simulink model "three_back_forth"  (R2023a)
settings: Solver=ode5  StartTime=0.0  StopTime=inf  FixedStep=0.001  RelTol=1e-3
undefined symbols (not defined in the file or in its folder): LF
libraries: instrumentseriallib x9, sldrtlib x1
settings Model: Creator=DELL  LastModifiedBy=DELL
settings HardwareCC: ProdBitPerLong=64  ProdHWDeviceType=Intel->x86-64 (Linux 64)
settings ModelReferenceCC: EnableRefExpFcnMdlSchedulingChecks=on
settings RTWCC: Description=Simulink Desktop Real-Time  SystemTargetFile=sldrt.tlc  TemplateMakefile=sldrt.tmf  RTWCompilerOptimization=on
settings CodeAppCC: MaxIdLength=95
settings SimulinkDesktopRealTimeCC: TargetLibSuffix=_sldrt.a  TargetPreCompLibLocation=C:\Program Files\MATLAB\R2023a\toolbox\sldrt\lib\win64

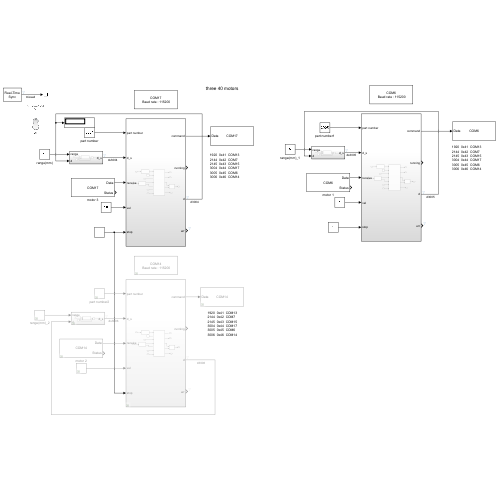
[thumbnail: Simulink's stored preview of the top-level diagram]
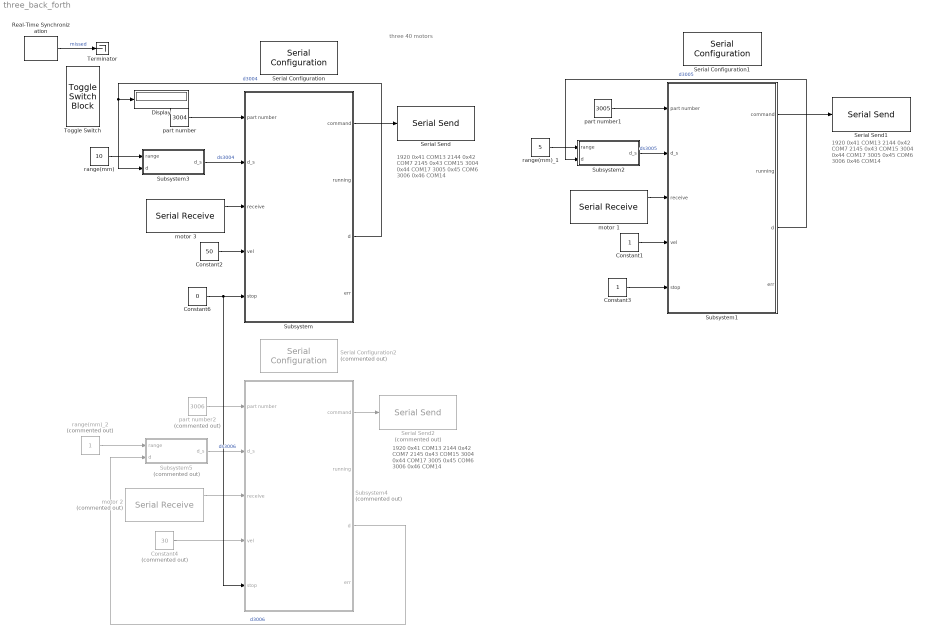
== system three_back_forth ==
  note: 1920  0x41  COM13
      | 2144  0x42  COM7
      | 2145  0x43  COM15
      | 3004  0x44  COM17
      | 3005  0x45  COM6
      | 3006  0x46  COM14
  note: 1920  0x41  COM13
      | 2144  0x42  COM7
      | 2145  0x43  COM15
      | 3004  0x44  COM17
      | 3005  0x45  COM6
      | 3006  0x46  COM14
  note: 1920  0x41  COM13
      | 2144  0x42  COM7
      | 2145  0x43  COM15
      | 3004  0x44  COM17
      | 3005  0x45  COM6
      | 3006  0x46  COM14
  note: three 40 motors
  Constant1 : Constant
  Constant2 : Constant  Value=50
  Constant3 : Constant
  Constant4 : Constant  Commented=on  Value=30
  Constant6 : Constant  Value=0
  Display : Display
  Real-Time Synchronization : sldrtlib/Real-Time Synchronization  SampleTime=0.1  MaxMissedTicks=10  ShowMissedTicks=on  YieldWhenWaiting=off
  Serial Configuration : instrumentseriallib/Serial Configuration  Priority=-200000  PortSel=COM17  Port=COM17  ComPort=COM17  BaudRate=115200  DataBits=8  Parity=none  StopBits=1  ByteOrder=little-endian  FlowControl=none  Timeout=10  SimulateUsing=Interpreted execution  BlockInModel=on  aMode=1
  Serial Configuration1 : instrumentseriallib/Serial Configuration  Priority=-200000  PortSel=COM6  Port=COM6  ComPort=COM6  BaudRate=115200  DataBits=8  Parity=none  StopBits=1  ByteOrder=little-endian  FlowControl=none  Timeout=10  SimulateUsing=Interpreted execution  BlockInModel=on  aMode=1
  Serial Configuration2 : instrumentseriallib/Serial Configuration  Priority=-200000  Commented=on  PortSel=COM14  Port=COM14  ComPort=COM14  BaudRate=115200  DataBits=8  Parity=none  StopBits=1  ByteOrder=little-endian  FlowControl=none  Timeout=10  SimulateUsing=Interpreted execution  BlockInModel=on  aMode=1
  Serial Send : instrumentseriallib/Serial Send  Priority=1  PortSel=COM17  Port=COM17  ComPort=COM17  Header=[]  Terminator=<none>  CustomTerminator=[]  EnableBlockingMode=off  SimulateUsing=Interpreted execution  BlockInModel=on  aMode=1
  Serial Send1 : instrumentseriallib/Serial Send  Priority=1  PortSel=COM6  Port=COM6  ComPort=COM6  Header=[]  Terminator=<none>  CustomTerminator=[]  EnableBlockingMode=off  SimulateUsing=Interpreted execution  BlockInModel=on  aMode=1
  Serial Send2 : instrumentseriallib/Serial Send  Priority=1  Commented=on  PortSel=COM14  Port=COM14  ComPort=COM14  Header=[]  Terminator=<none>  CustomTerminator=[]  EnableBlockingMode=off  SimulateUsing=Interpreted execution  BlockInModel=on  aMode=1
  Subsystem : Subsystem
  Subsystem1 : Subsystem
  Subsystem2 : Subsystem
  Subsystem3 : Subsystem
  Subsystem4 : Subsystem  Commented=on
  Subsystem5 : Subsystem  Commented=on
  Terminator : Terminator
  Toggle Switch : ToggleSwitchBlock
      settings: Values={{'Off', 'On'}, [0 1]}
  motor 1 : instrumentseriallib/Serial Receive  Priority=1  PortSel=COM6  Port=COM6  ComPort=COM6  DataType=uint8  SaveDataType=uint8  ToggleHeader=off  Header=[]  ToggleTerminator=on  Terminator=LF ('\n')  CustomTerminator=[]  InputFormat=Column major  ToggleDataSize=on  DataSize=[1 7]  EnableBlockingMode=off  ActionDataUnavailable=Output last received value  ActionWhenDataUnavailable=Output last received value  CustomValue=0  SampleTime=0.01  SimulateUsing=Interpreted execution  BlockInModel=on  aMode=1
  motor 2 : instrumentseriallib/Serial Receive  Priority=1  Commented=on  PortSel=COM14  Port=COM14  ComPort=COM14  DataType=uint8  SaveDataType=uint8  ToggleHeader=off  Header=[]  ToggleTerminator=on  Terminator=LF ('\n')  CustomTerminator=[]  InputFormat=Column major  ToggleDataSize=on  DataSize=[1 7]  EnableBlockingMode=off  ActionDataUnavailable=Output last received value  ActionWhenDataUnavailable=Output last received value  CustomValue=0  SampleTime=0.01  SimulateUsing=Interpreted execution  BlockInModel=on  aMode=1
  motor 3 : instrumentseriallib/Serial Receive  Priority=1  PortSel=COM17  Port=COM17  ComPort=COM17  DataType=uint8  SaveDataType=uint8  ToggleHeader=off  Header=[]  ToggleTerminator=on  Terminator=LF ('\n')  CustomTerminator=[]  InputFormat=Column major  ToggleDataSize=on  DataSize=[1 7]  EnableBlockingMode=off  ActionDataUnavailable=Output last received value  ActionWhenDataUnavailable=Output last received value  CustomValue=0  SampleTime=0.01  SimulateUsing=Interpreted execution  BlockInModel=on  aMode=1
  part number : Constant  Value=3004
  part number1 : Constant  Value=3005
  part number2 : Constant  Commented=on  Value=3006
  range(mm) : Constant  Value=10
  range(mm)_1 : Constant  Value=5
  range(mm)_2 : Constant  Commented=on
  wires:
  range(mm)/1 -> Subsystem3/1(range)
  part number/1 -> Subsystem/1(part number)
  Subsystem3/1(d_s) -> Subsystem/2(d_s)  "ds3004"
  motor 3/1 -> Subsystem/3(receive)
  Subsystem/1(command) -> Serial Send/1
  Subsystem/3(d) -> Display/1, Subsystem3/2(d)  "d3004"
  Constant2/1 -> Subsystem/4(vel)
  Subsystem1/1(command) -> Serial Send1/1
  Constant1/1 -> Subsystem1/4(vel)
  part number1/1 -> Subsystem1/1(part number)
  motor 1/1 -> Subsystem1/3(receive)
  Subsystem2/1(d_s) -> Subsystem1/2(d_s)  "ds3005"
  range(mm)_1/1 -> Subsystem2/1(range)
  Subsystem1/3(d) -> Subsystem2/2(d)  "d3005"
  Subsystem4/1(command) -> Serial Send2/1
  Constant4/1 -> Subsystem4/4(vel)
  part number2/1 -> Subsystem4/1(part number)
  motor 2/1 -> Subsystem4/3(receive)
  Subsystem5/1(d_s) -> Subsystem4/2(d_s)  "ds3006"
  range(mm)_2/1 -> Subsystem5/1(range)
  Subsystem4/3(d) -> Subsystem5/2(d)  "d3006"
  Real-Time Synchronization/1 -> Terminator/1  "missed"
  Constant6/1 -> Subsystem4/5(stop), Subsystem/5(stop)
  Constant3/1 -> Subsystem1/5(stop)

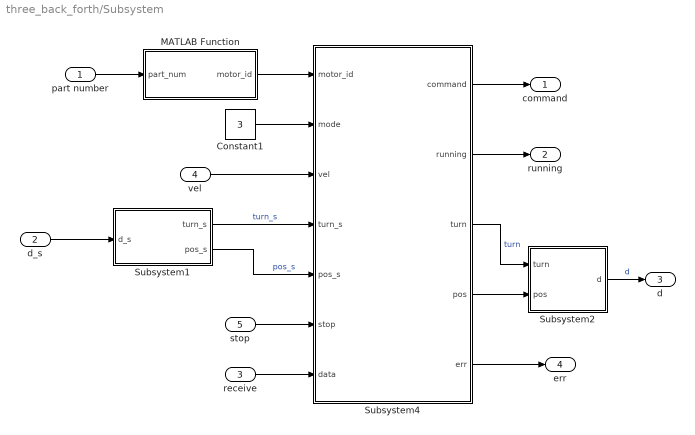
== system three_back_forth/Subsystem ==
  part number : Inport
  d_s : Inport  Port=2
  receive : Inport  Port=3
  vel : Inport  Port=4
  stop : Inport  Port=5
  Constant1 : Constant  Value=3
  MATLAB Function : MATLAB Function  TreatAsAtomicUnit=on
  Subsystem1 : Subsystem
  Subsystem2 : Subsystem
  Subsystem4 : Subsystem
  command : Outport
  running : Outport  Port=2
  d : Outport  Port=3
  err : Outport  Port=4
  wires:
  Constant1/1 -> Subsystem4/2(mode)
  Subsystem4/2(running) -> running/1
  Subsystem1/1(turn_s) -> Subsystem4/4(turn_s)  "turn_s"
  Subsystem1/2(pos_s) -> Subsystem4/5(pos_s)  "pos_s"
  Subsystem4/3(turn) -> Subsystem2/1(turn)  "turn"
  Subsystem4/1(command) -> command/1
  Subsystem4/4(pos) -> Subsystem2/2(pos)
  vel/1 -> Subsystem4/3(vel)
  stop/1 -> Subsystem4/6(stop)
  receive/1 -> Subsystem4/7(data)
  part number/1 -> MATLAB Function/1(part_num)
  Subsystem2/1(d) -> d/1  "d"
  d_s/1 -> Subsystem1/1(d_s)
  Subsystem4/5(err) -> err/1
  MATLAB Function/1(motor_id) -> Subsystem4/1(motor_id)

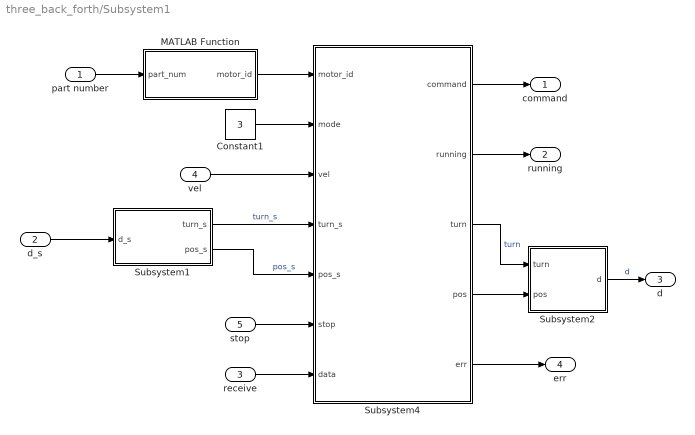
== system three_back_forth/Subsystem1 ==
  part number : Inport
  d_s : Inport  Port=2
  receive : Inport  Port=3
  vel : Inport  Port=4
  stop : Inport  Port=5
  Constant1 : Constant  Value=3
  MATLAB Function : MATLAB Function  TreatAsAtomicUnit=on
  Subsystem1 : Subsystem
  Subsystem2 : Subsystem
  Subsystem4 : Subsystem
  command : Outport
  running : Outport  Port=2
  d : Outport  Port=3
  err : Outport  Port=4
  wires:
  Constant1/1 -> Subsystem4/2(mode)
  Subsystem4/2(running) -> running/1
  Subsystem1/1(turn_s) -> Subsystem4/4(turn_s)  "turn_s"
  Subsystem1/2(pos_s) -> Subsystem4/5(pos_s)  "pos_s"
  Subsystem4/3(turn) -> Subsystem2/1(turn)  "turn"
  Subsystem4/1(command) -> command/1
  Subsystem4/4(pos) -> Subsystem2/2(pos)
  vel/1 -> Subsystem4/3(vel)
  stop/1 -> Subsystem4/6(stop)
  receive/1 -> Subsystem4/7(data)
  part number/1 -> MATLAB Function/1(part_num)
  Subsystem2/1(d) -> d/1  "d"
  d_s/1 -> Subsystem1/1(d_s)
  Subsystem4/5(err) -> err/1
  MATLAB Function/1(motor_id) -> Subsystem4/1(motor_id)

== system three_back_forth/Subsystem2 ==
  range : Inport
  d : Inport  Port=2
  Constant : Constant  Value=0.001
  MATLAB System : MATLABSystem  System=toggle_system  SimulateUsing=Code generation
      mask Type: toggle_system
      mask Display:
      | disp('toggle_system');
      | port_label('input',1,'range');
      | port_label('input',2,'d');
      | port_label('input',3,'margin');
      | port_label('output',1,'toggle');
  Product : Product
  d_s : Outport
  wires:
  d/1 -> MATLAB System/2
  range/1 -> Product/2, MATLAB System/1
  MATLAB System/1 -> Product/1
  Product/1 -> d_s/1
  Constant/1 -> MATLAB System/3

== system three_back_forth/Subsystem3 ==
  range : Inport
  d : Inport  Port=2
  Constant : Constant  Value=0.001
  MATLAB System : MATLABSystem  System=toggle_system  SimulateUsing=Code generation
      mask Type: toggle_system
      mask Display:
      | disp('toggle_system');
      | port_label('input',1,'range');
      | port_label('input',2,'d');
      | port_label('input',3,'margin');
      | port_label('output',1,'toggle');
  Product : Product
  d_s : Outport
  wires:
  d/1 -> MATLAB System/2
  range/1 -> Product/2, MATLAB System/1
  MATLAB System/1 -> Product/1
  Product/1 -> d_s/1
  Constant/1 -> MATLAB System/3

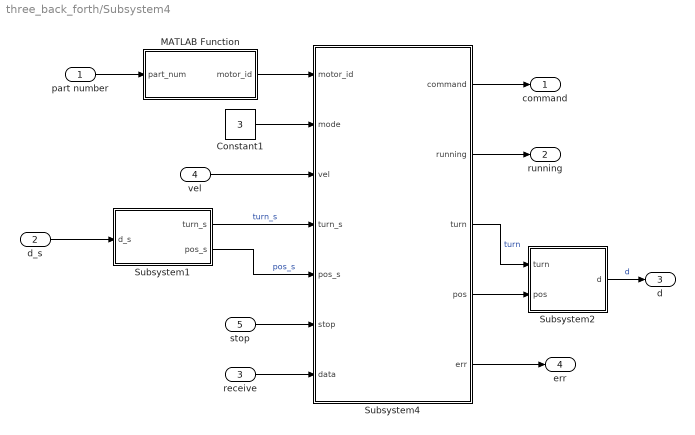
== system three_back_forth/Subsystem4 ==
  part number : Inport
  d_s : Inport  Port=2
  receive : Inport  Port=3
  vel : Inport  Port=4
  stop : Inport  Port=5
  Constant1 : Constant  Value=3
  MATLAB Function : MATLAB Function  TreatAsAtomicUnit=on
  Subsystem1 : Subsystem
  Subsystem2 : Subsystem
  Subsystem4 : Subsystem
  command : Outport
  running : Outport  Port=2
  d : Outport  Port=3
  err : Outport  Port=4
  wires:
  Constant1/1 -> Subsystem4/2(mode)
  Subsystem4/2(running) -> running/1
  Subsystem1/1(turn_s) -> Subsystem4/4(turn_s)  "turn_s"
  Subsystem1/2(pos_s) -> Subsystem4/5(pos_s)  "pos_s"
  Subsystem4/3(turn) -> Subsystem2/1(turn)  "turn"
  Subsystem4/1(command) -> command/1
  Subsystem4/4(pos) -> Subsystem2/2(pos)
  vel/1 -> Subsystem4/3(vel)
  stop/1 -> Subsystem4/6(stop)
  receive/1 -> Subsystem4/7(data)
  part number/1 -> MATLAB Function/1(part_num)
  Subsystem2/1(d) -> d/1  "d"
  d_s/1 -> Subsystem1/1(d_s)
  Subsystem4/5(err) -> err/1
  MATLAB Function/1(motor_id) -> Subsystem4/1(motor_id)

== system three_back_forth/Subsystem5 ==
  range : Inport
  d : Inport  Port=2
  Constant : Constant  Value=0.001
  MATLAB System : MATLABSystem  System=toggle_system  SimulateUsing=Code generation
      mask Type: toggle_system
      mask Display:
      | disp('toggle_system');
      | port_label('input',1,'range');
      | port_label('input',2,'d');
      | port_label('input',3,'margin');
      | port_label('output',1,'toggle');
  Product : Product
  d_s : Outport
  wires:
  d/1 -> MATLAB System/2
  range/1 -> Product/2, MATLAB System/1
  MATLAB System/1 -> Product/1
  Product/1 -> d_s/1
  Constant/1 -> MATLAB System/3

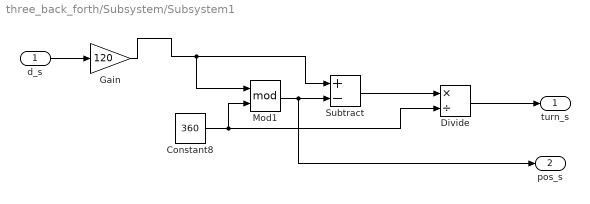
== system three_back_forth/Subsystem/Subsystem1 ==
  d_s : Inport
  Constant8 : Constant  Value=360
  Divide : Product  Inputs=*/
  Gain : Gain  Gain=120
  Mod1 : Math  Operator=mod
  Subtract : Sum  Inputs=+-
  turn_s : Outport
  pos_s : Outport  Port=2
  wires:
  Constant8/1 -> Divide/2, Mod1/2
  Gain/1 -> Subtract/1, Mod1/1
  Mod1/1 -> pos_s/1, Subtract/2
  Subtract/1 -> Divide/1
  Divide/1 -> turn_s/1
  d_s/1 -> Gain/1

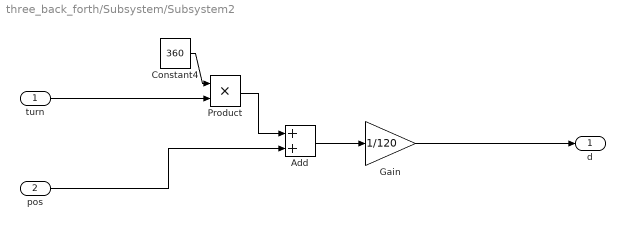
== system three_back_forth/Subsystem/Subsystem2 ==
  turn : Inport
  pos : Inport  Port=2
  Add : Sum
  Constant4 : Constant  Value=360
  Gain : Gain  Gain=1/120
  Product : Product
  d : Outport
  wires:
  turn/1 -> Product/2
  Add/1 -> Gain/1
  Constant4/1 -> Product/1
  Product/1 -> Add/1
  Gain/1 -> d/1
  pos/1 -> Add/2

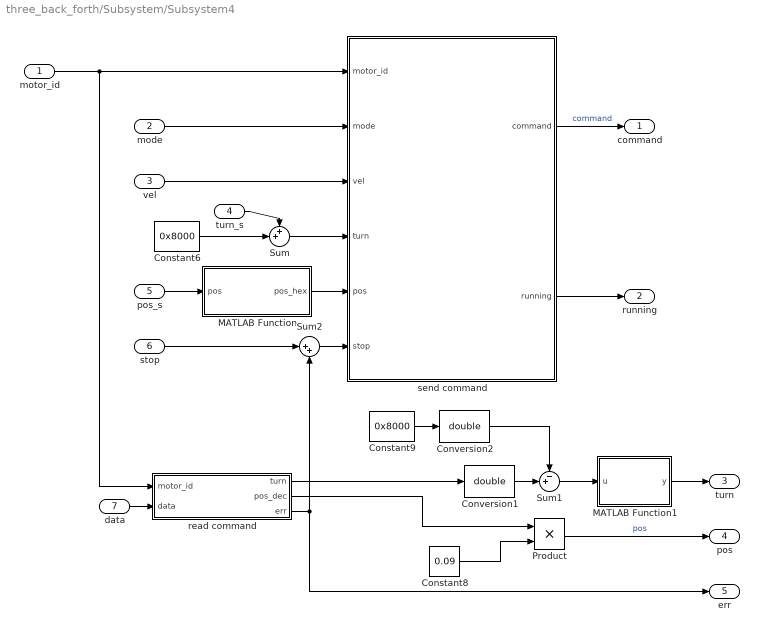
== system three_back_forth/Subsystem/Subsystem4 ==
  motor_id : Inport
  mode : Inport  Port=2
  vel : Inport  Port=3
  turn_s : Inport  Port=4
  pos_s : Inport  Port=5
  stop : Inport  Port=6
  data : Inport  Port=7
  Constant6 : Constant  Value=0x8000
  Constant8 : Constant  Value=0.09
  Constant9 : Constant  Value=0x8000
  Conversion1 : DataTypeConversion  OutDataTypeStr=double  SaturateOnIntegerOverflow=off  RndMeth=Floor
  Conversion2 : DataTypeConversion  OutDataTypeStr=double  SaturateOnIntegerOverflow=off  RndMeth=Floor
  MATLAB Function : MATLAB Function  TreatAsAtomicUnit=on
  MATLAB Function1 : MATLAB Function  TreatAsAtomicUnit=on
  Product : Product
  Sum : Sum  Inputs=++|
  Sum1 : Sum  Inputs=-+|
  Sum2 : Sum  Inputs=|++
  read command : MATLAB Function  TreatAsAtomicUnit=on
  send command : MATLAB Function  TreatAsAtomicUnit=on
  command : Outport
  running : Outport  Port=2
  turn : Outport  Port=3
  pos : Outport  Port=4
  err : Outport  Port=5
  wires:
  Constant6/1 -> Sum/2
  send command/2(running) -> running/1
  MATLAB Function/1(pos_hex) -> send command/5(pos)
  vel/1 -> send command/3(vel)
  read command/2(pos_dec) -> Product/1
  Sum/1 -> send command/4(turn)
  Constant8/1 -> Product/2
  Product/1 -> pos/1  "pos"
  data/1 -> read command/2(data)
  motor_id/1 -> read command/1(motor_id), send command/1(motor_id)
  send command/1(command) -> command/1  "command"
  pos_s/1 -> MATLAB Function/1(pos)
  mode/1 -> send command/2(mode)
  turn_s/1 -> Sum/1
  read command/1(turn) -> Conversion1/1
  Conversion1/1 -> Sum1/2
  Constant9/1 -> Conversion2/1
  Conversion2/1 -> Sum1/1
  Sum1/1 -> MATLAB Function1/1(u)
  MATLAB Function1/1(y) -> turn/1
  read command/3(err) -> err/1, Sum2/2
  stop/1 -> Sum2/1
  Sum2/1 -> send command/6(stop)

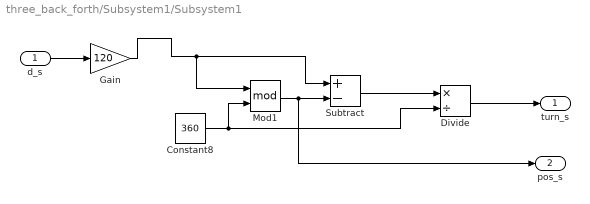
== system three_back_forth/Subsystem1/Subsystem1 ==
  d_s : Inport
  Constant8 : Constant  Value=360
  Divide : Product  Inputs=*/
  Gain : Gain  Gain=120
  Mod1 : Math  Operator=mod
  Subtract : Sum  Inputs=+-
  turn_s : Outport
  pos_s : Outport  Port=2
  wires:
  Constant8/1 -> Divide/2, Mod1/2
  Gain/1 -> Subtract/1, Mod1/1
  Mod1/1 -> pos_s/1, Subtract/2
  Subtract/1 -> Divide/1
  Divide/1 -> turn_s/1
  d_s/1 -> Gain/1

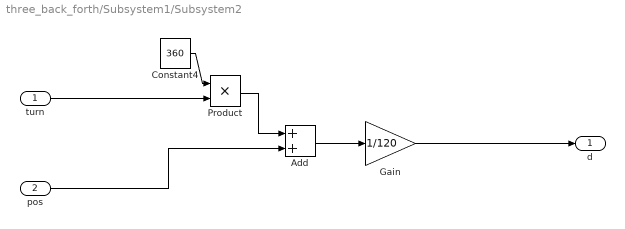
== system three_back_forth/Subsystem1/Subsystem2 ==
  turn : Inport
  pos : Inport  Port=2
  Add : Sum
  Constant4 : Constant  Value=360
  Gain : Gain  Gain=1/120
  Product : Product
  d : Outport
  wires:
  turn/1 -> Product/2
  Add/1 -> Gain/1
  Constant4/1 -> Product/1
  Product/1 -> Add/1
  Gain/1 -> d/1
  pos/1 -> Add/2

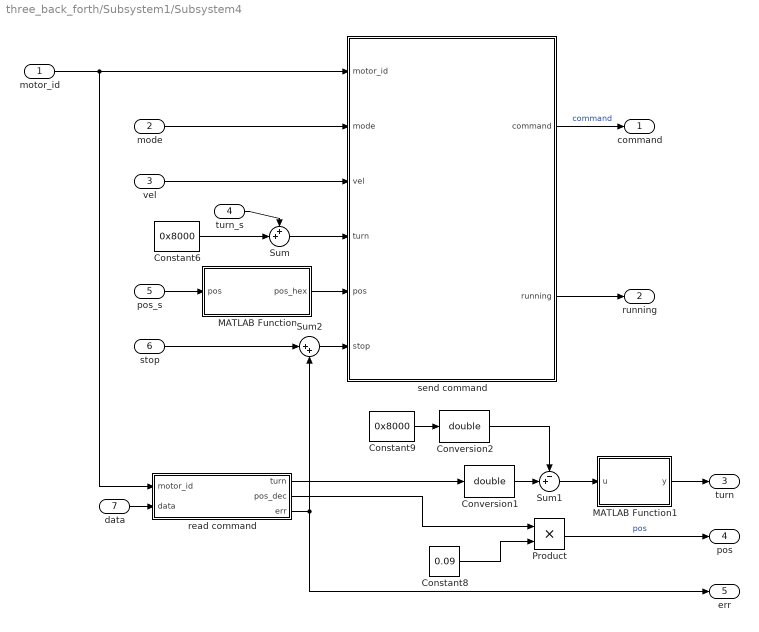
== system three_back_forth/Subsystem1/Subsystem4 ==
  motor_id : Inport
  mode : Inport  Port=2
  vel : Inport  Port=3
  turn_s : Inport  Port=4
  pos_s : Inport  Port=5
  stop : Inport  Port=6
  data : Inport  Port=7
  Constant6 : Constant  Value=0x8000
  Constant8 : Constant  Value=0.09
  Constant9 : Constant  Value=0x8000
  Conversion1 : DataTypeConversion  OutDataTypeStr=double  SaturateOnIntegerOverflow=off  RndMeth=Floor
  Conversion2 : DataTypeConversion  OutDataTypeStr=double  SaturateOnIntegerOverflow=off  RndMeth=Floor
  MATLAB Function : MATLAB Function  TreatAsAtomicUnit=on
  MATLAB Function1 : MATLAB Function  TreatAsAtomicUnit=on
  Product : Product
  Sum : Sum  Inputs=++|
  Sum1 : Sum  Inputs=-+|
  Sum2 : Sum  Inputs=|++
  read command : MATLAB Function  TreatAsAtomicUnit=on
  send command : MATLAB Function  TreatAsAtomicUnit=on
  command : Outport
  running : Outport  Port=2
  turn : Outport  Port=3
  pos : Outport  Port=4
  err : Outport  Port=5
  wires:
  Constant6/1 -> Sum/2
  send command/2(running) -> running/1
  MATLAB Function/1(pos_hex) -> send command/5(pos)
  vel/1 -> send command/3(vel)
  read command/2(pos_dec) -> Product/1
  Sum/1 -> send command/4(turn)
  Constant8/1 -> Product/2
  Product/1 -> pos/1  "pos"
  data/1 -> read command/2(data)
  motor_id/1 -> read command/1(motor_id), send command/1(motor_id)
  send command/1(command) -> command/1  "command"
  pos_s/1 -> MATLAB Function/1(pos)
  mode/1 -> send command/2(mode)
  turn_s/1 -> Sum/1
  read command/1(turn) -> Conversion1/1
  Conversion1/1 -> Sum1/2
  Constant9/1 -> Conversion2/1
  Conversion2/1 -> Sum1/1
  Sum1/1 -> MATLAB Function1/1(u)
  MATLAB Function1/1(y) -> turn/1
  read command/3(err) -> err/1, Sum2/2
  stop/1 -> Sum2/1
  Sum2/1 -> send command/6(stop)

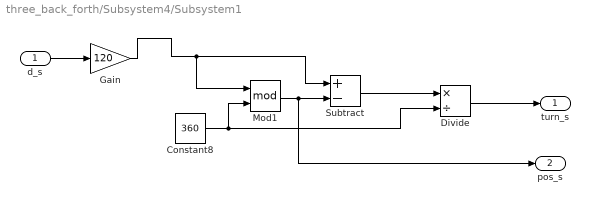
== system three_back_forth/Subsystem4/Subsystem1 ==
  d_s : Inport
  Constant8 : Constant  Value=360
  Divide : Product  Inputs=*/
  Gain : Gain  Gain=120
  Mod1 : Math  Operator=mod
  Subtract : Sum  Inputs=+-
  turn_s : Outport
  pos_s : Outport  Port=2
  wires:
  Constant8/1 -> Divide/2, Mod1/2
  Gain/1 -> Subtract/1, Mod1/1
  Mod1/1 -> pos_s/1, Subtract/2
  Subtract/1 -> Divide/1
  Divide/1 -> turn_s/1
  d_s/1 -> Gain/1

== system three_back_forth/Subsystem4/Subsystem2 ==
  turn : Inport
  pos : Inport  Port=2
  Add : Sum
  Constant4 : Constant  Value=360
  Gain : Gain  Gain=1/120
  Product : Product
  d : Outport
  wires:
  turn/1 -> Product/2
  Add/1 -> Gain/1
  Constant4/1 -> Product/1
  Product/1 -> Add/1
  Gain/1 -> d/1
  pos/1 -> Add/2

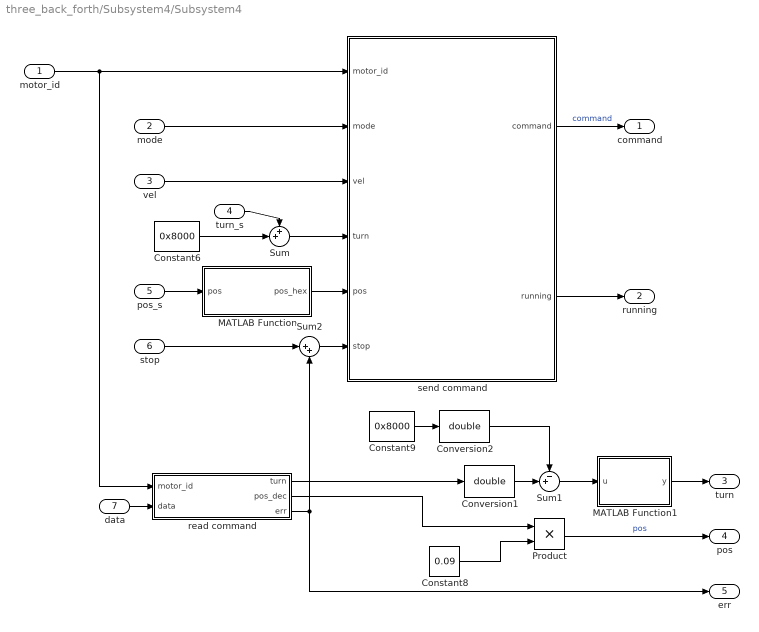
== system three_back_forth/Subsystem4/Subsystem4 ==
  motor_id : Inport
  mode : Inport  Port=2
  vel : Inport  Port=3
  turn_s : Inport  Port=4
  pos_s : Inport  Port=5
  stop : Inport  Port=6
  data : Inport  Port=7
  Constant6 : Constant  Value=0x8000
  Constant8 : Constant  Value=0.09
  Constant9 : Constant  Value=0x8000
  Conversion1 : DataTypeConversion  OutDataTypeStr=double  SaturateOnIntegerOverflow=off  RndMeth=Floor
  Conversion2 : DataTypeConversion  OutDataTypeStr=double  SaturateOnIntegerOverflow=off  RndMeth=Floor
  MATLAB Function : MATLAB Function  TreatAsAtomicUnit=on
  MATLAB Function1 : MATLAB Function  TreatAsAtomicUnit=on
  Product : Product
  Sum : Sum  Inputs=++|
  Sum1 : Sum  Inputs=-+|
  Sum2 : Sum  Inputs=|++
  read command : MATLAB Function  TreatAsAtomicUnit=on
  send command : MATLAB Function  TreatAsAtomicUnit=on
  command : Outport
  running : Outport  Port=2
  turn : Outport  Port=3
  pos : Outport  Port=4
  err : Outport  Port=5
  wires:
  Constant6/1 -> Sum/2
  send command/2(running) -> running/1
  MATLAB Function/1(pos_hex) -> send command/5(pos)
  vel/1 -> send command/3(vel)
  read command/2(pos_dec) -> Product/1
  Sum/1 -> send command/4(turn)
  Constant8/1 -> Product/2
  Product/1 -> pos/1  "pos"
  data/1 -> read command/2(data)
  motor_id/1 -> read command/1(motor_id), send command/1(motor_id)
  send command/1(command) -> command/1  "command"
  pos_s/1 -> MATLAB Function/1(pos)
  mode/1 -> send command/2(mode)
  turn_s/1 -> Sum/1
  read command/1(turn) -> Conversion1/1
  Conversion1/1 -> Sum1/2
  Constant9/1 -> Conversion2/1
  Conversion2/1 -> Sum1/1
  Sum1/1 -> MATLAB Function1/1(u)
  MATLAB Function1/1(y) -> turn/1
  read command/3(err) -> err/1, Sum2/2
  stop/1 -> Sum2/1
  Sum2/1 -> send command/6(stop)

== matlab function three_back_forth/Subsystem4/MATLAB Function ==
  data: part_num input; motor_id output
function motor_id = motor_id(part_num)
    motor_id=0x40;
    switch part_num
        case 1920
            motor_id=0x41;
        case 2144
            motor_id=0x42;
        case 2145
            motor_id=0x43;
        case 3004
            motor_id = 0x44;
        case 3005
            motor_id = 0x45;
        case 3006
            motor_id = 0x46;
        otherwise
            motor_id = 0x40;
    end
end

== matlab function three_back_forth/Subsystem4/Subsystem4/MATLAB Function ==
  data: pos input; pos_hex output
function pos_hex = fcn(pos)
pos = pos/0.09;
pos_hex = 0x0000;
mult = 1;
while pos>0
    digit = mod(pos,10);
    pos = pos - digit;
    pos = pos/10;
    pos_hex = pos_hex + uint16(mult*digit);
    mult = mult*16;
end

== matlab function three_back_forth/Subsystem4/Subsystem4/MATLAB Function1 ==
  data: u input; y output
function y = adjust_init(u)
if(u<=-32767)
    y=0;
else
    y = u;
end

== matlab function three_back_forth/Subsystem4/Subsystem4/read command ==
  data: motor_id input; data input; turn output; pos_dec output; err output
function [turn,pos_dec,err] = fcn(motor_id, data)
err=0;
turn=0x8000;
pos_dec=0x0000;
if data(1)~=motor_id
    err=1;
    return
end
if data(2)~=0x54
    err=2;
    return
end
turn = uint16(data(3))*0x100 + uint16(data(4));
pos = uint16(data(5))*0x100 + uint16(data(6));
pos_dec = 0x0000;
mult = 1;
while pos>0
    p1 = mod(pos,0x0010);
    pos = pos - p1;
    pos = pos/0x0010;
    pos_dec = pos_dec + p1*mult;
    mult = mult*10;
end

== matlab function three_back_forth/Subsystem4/Subsystem4/send command ==
  data: motor_id input; mode input; vel input; command output; turn input; running output; pos input; stop input
function [command ,running]= fcn(motor_id, mode, vel,turn,pos,stop)
    command = uint8(zeros(1,16));
    command(9:16) = [motor_id 0x51 0 0 0 0 0 0x0A];

    command(8) = 0x0A;
    command(1) = motor_id;
    running = 1;
    % force stop
    if  stop == 1
        command(2) = 0x53;       
        running = 0;
        return        
    end

    % set mode
    switch mode
        % continues velocity loop
        case 1
            if vel>0
                command(2) = 0x44;
            elseif vel<0
                command(2)=0x55;   
            else
                command(2) = 0x53;
                running = 0;   
            end
            command(7) = abs(vel);
        % impulse velocity loop
        case 2
            if vel>0
                command(2) = 0x46;
            elseif vel<0
                command(2)=0x56;  
            else
                command(2) = 0x53;
                running = 0;                   
            end
            command(7) = abs(vel);
        % coontinue position loop
        case 3
            command(2) = 2;
            command(3) = uint8((turn-mod(turn,0x100))/0x100);
            command(4) = uint8(mod(turn,0x100));
            command(5) = uint8((pos-mod(pos,0x100))/0x100);
            command(6) = uint8(mod(pos,0x100));            
            command(7) = abs(vel);
        % impulse position loop
        case 4
            command(2) = 3;
            command(3) = uint8((turn-mod(turn,0x100))/0x100);
            command(4) = uint8(mod(turn,0x100));
            command(5) = uint8((pos-mod(pos,0x100))/0x100);
            command(6) = uint8(mod(pos,0x100));                
            command(7) = abs(vel);
        case 5
            command(2) = 0x52;
        otherwise
            command(2) = 0x53;       
            running = 0;
    end
end

== matlab function three_back_forth/Subsystem/MATLAB Function ==
  data: part_num input; motor_id output
function motor_id = motor_id(part_num)
    motor_id=0x40;
    switch part_num
        case 1920
            motor_id=0x41;
        case 2144
            motor_id=0x42;
        case 2145
            motor_id=0x43;
        case 3004
            motor_id = 0x44;
        case 3005
            motor_id = 0x45;
        case 3006
            motor_id = 0x46;
        otherwise
            motor_id = 0x40;
    end
end

== matlab function three_back_forth/Subsystem1/MATLAB Function ==
  data: part_num input; motor_id output
function motor_id = motor_id(part_num)
    motor_id=0x40;
    switch part_num
        case 1920
            motor_id=0x41;
        case 2144
            motor_id=0x42;
        case 2145
            motor_id=0x43;
        case 3004
            motor_id = 0x44;
        case 3005
            motor_id = 0x45;
        case 3006
            motor_id = 0x46;
        otherwise
            motor_id = 0x40;
    end
end

== matlab function three_back_forth/Subsystem1/Subsystem4/MATLAB Function ==
  data: pos input; pos_hex output
function pos_hex = fcn(pos)
pos = pos/0.09;
pos_hex = 0x0000;
mult = 1;
while pos>0
    digit = mod(pos,10);
    pos = pos - digit;
    pos = pos/10;
    pos_hex = pos_hex + uint16(mult*digit);
    mult = mult*16;
end

== matlab function three_back_forth/Subsystem1/Subsystem4/MATLAB Function1 ==
  data: u input; y output
function y = adjust_init(u)
if(u<=-32767)
    y=0;
else
    y = u;
end

== matlab function three_back_forth/Subsystem/Subsystem4/MATLAB Function ==
  data: pos input; pos_hex output
function pos_hex = fcn(pos)
pos = pos/0.09;
pos_hex = 0x0000;
mult = 1;
while pos>0
    digit = mod(pos,10);
    pos = pos - digit;
    pos = pos/10;
    pos_hex = pos_hex + uint16(mult*digit);
    mult = mult*16;
end

== matlab function three_back_forth/Subsystem/Subsystem4/MATLAB Function1 ==
  data: u input; y output
function y = adjust_init(u)
if(u<=-32767)
    y=0;
else
    y = u;
end

== matlab function three_back_forth/Subsystem/Subsystem4/read command ==
  data: motor_id input; data input; turn output; pos_dec output; err output
function [turn,pos_dec,err] = fcn(motor_id, data)
err=0;
turn=0x8000;
pos_dec=0x0000;
if data(1)~=motor_id
    err=1;
    return
end
if data(2)~=0x54
    err=2;
    return
end
turn = uint16(data(3))*0x100 + uint16(data(4));
pos = uint16(data(5))*0x100 + uint16(data(6));
pos_dec = 0x0000;
mult = 1;
while pos>0
    p1 = mod(pos,0x0010);
    pos = pos - p1;
    pos = pos/0x0010;
    pos_dec = pos_dec + p1*mult;
    mult = mult*10;
end

== matlab function three_back_forth/Subsystem/Subsystem4/send command ==
  data: motor_id input; mode input; vel input; command output; turn input; running output; pos input; stop input
function [command ,running]= fcn(motor_id, mode, vel,turn,pos,stop)
    command = uint8(zeros(1,16));
    command(9:16) = [motor_id 0x51 0 0 0 0 0 0x0A];

    command(8) = 0x0A;
    command(1) = motor_id;
    running = 1;
    % force stop
    if  stop == 1
        command(2) = 0x53;       
        running = 0;
        return        
    end

    % set mode
    switch mode
        % continues velocity loop
        case 1
            if vel>0
                command(2) = 0x44;
            elseif vel<0
                command(2)=0x55;   
            else
                command(2) = 0x53;
                running = 0;   
            end
            command(7) = abs(vel);
        % impulse velocity loop
        case 2
            if vel>0
                command(2) = 0x46;
            elseif vel<0
                command(2)=0x56;  
            else
                command(2) = 0x53;
                running = 0;                   
            end
            command(7) = abs(vel);
        % coontinue position loop
        case 3
            command(2) = 2;
            command(3) = uint8((turn-mod(turn,0x100))/0x100);
            command(4) = uint8(mod(turn,0x100));
            command(5) = uint8((pos-mod(pos,0x100))/0x100);
            command(6) = uint8(mod(pos,0x100));            
            command(7) = abs(vel);
        % impulse position loop
        case 4
            command(2) = 3;
            command(3) = uint8((turn-mod(turn,0x100))/0x100);
            command(4) = uint8(mod(turn,0x100));
            command(5) = uint8((pos-mod(pos,0x100))/0x100);
            command(6) = uint8(mod(pos,0x100));                
            command(7) = abs(vel);
        case 5
            command(2) = 0x52;
        otherwise
            command(2) = 0x53;       
            running = 0;
    end
end

== matlab function three_back_forth/Subsystem1/Subsystem4/read command ==
  data: motor_id input; data input; turn output; pos_dec output; err output
function [turn,pos_dec,err] = fcn(motor_id, data)
err=0;
turn=0x8000;
pos_dec=0x0000;
if data(1)~=motor_id
    err=1;
    return
end
if data(2)~=0x54
    err=2;
    return
end
turn = uint16(data(3))*0x100 + uint16(data(4));
pos = uint16(data(5))*0x100 + uint16(data(6));
pos_dec = 0x0000;
mult = 1;
while pos>0
    p1 = mod(pos,0x0010);
    pos = pos - p1;
    pos = pos/0x0010;
    pos_dec = pos_dec + p1*mult;
    mult = mult*10;
end

== matlab function three_back_forth/Subsystem1/Subsystem4/send command ==
  data: motor_id input; mode input; vel input; command output; turn input; running output; pos input; stop input
function [command ,running]= fcn(motor_id, mode, vel,turn,pos,stop)
    command = uint8(zeros(1,16));
    command(9:16) = [motor_id 0x51 0 0 0 0 0 0x0A];

    command(8) = 0x0A;
    command(1) = motor_id;
    running = 1;
    % force stop
    if  stop == 1
        command(2) = 0x53;       
        running = 0;
        return        
    end

    % set mode
    switch mode
        % continues velocity loop
        case 1
            if vel>0
                command(2) = 0x44;
            elseif vel<0
                command(2)=0x55;   
            else
                command(2) = 0x53;
                running = 0;   
            end
            command(7) = abs(vel);
        % impulse velocity loop
        case 2
            if vel>0
                command(2) = 0x46;
            elseif vel<0
                command(2)=0x56;  
            else
                command(2) = 0x53;
                running = 0;                   
            end
            command(7) = abs(vel);
        % coontinue position loop
        case 3
            command(2) = 2;
            command(3) = uint8((turn-mod(turn,0x100))/0x100);
            command(4) = uint8(mod(turn,0x100));
            command(5) = uint8((pos-mod(pos,0x100))/0x100);
            command(6) = uint8(mod(pos,0x100));            
            command(7) = abs(vel);
        % impulse position loop
        case 4
            command(2) = 3;
            command(3) = uint8((turn-mod(turn,0x100))/0x100);
            command(4) = uint8(mod(turn,0x100));
            command(5) = uint8((pos-mod(pos,0x100))/0x100);
            command(6) = uint8(mod(pos,0x100));                
            command(7) = abs(vel);
        case 5
            command(2) = 0x52;
        otherwise
            command(2) = 0x53;       
            running = 0;
    end
end
